simulink model "sldemo_flipflop"  (R2019b)
settings: Solver=VariableStepDiscrete  StartTime=0.0  StopTime=100  RelTol=1e-3  AbsTol=1e-6
StartFcn:
  | set_param('sldemo_flipflop/Display/Scope','Open','on');
libraries: simulink_extras x3
Description:
  | Modulo-4 Counter Using Flip-Flops
  | 
  | This example shows how to use Flip-Flop blocks (found in the Simulink(R)
  | Extras Library) to implement a Modulo-4 counter. The model takes the output
  | of a Modulo-4 counter and generates a half clock cycle width pulse on every
  | fourth clock pulses. Effectively, it produces a pulse whenever both outputs
  | of the Modulo-4 counter are equal to 1.
settings Model: ExtModeTrigMode=oneshot  ExtModeArmWhenConnect=off  ExtModeAutoUpdateStatusClock=off  Creator=The MathWorks, Inc.  LastModifiedBy=The MathWorks, Inc.
settings SolverCC: AutoScaleAbsTol=off
settings DataIOCC: ExternalInput=[]  InitialState=[]  SaveFormat=Array  SaveOutput=off  SignalLogging=off  SaveTime=off
settings OptimizationCC: BlockReduction=off  InitFltsAndDblsToZero=on  LifeSpan=inf  BufferReusableBoundary=off
settings DebuggingCC: SaveWithParameterizedLinksMsg=none  UnderspecifiedInitializationDetection=Classic  MergeDetectMultiDrivingBlocksExec=none  SignalResolutionControl=TryResolveAllWithWarning  MultiTaskDSMMsg=warning  MultiTaskCondExecSysMsg=none  IntegerOverflowMsg=none  FcnCallInpInsideContextMsg=warning  UnconnectedOutputMsg=none  BusObjectLabelMismatch=none  StateNameClashWarn=warning  SFUnexpectedBacktrackingDiag=warning  SFNoUnconditionalDefaultTransitionDiag=warning  SFExecutionAtInitializationDiag=none  IntegerSaturationMsg=none  ArithmeticOperatorsInVariantConditions=warning
settings HardwareCC: ProdBitPerPointer=32  ProdBitPerSizeT=32  ProdBitPerPtrDiffT=32  ProdLargestAtomicFloat=None  ProdIntDivRoundTo=Undefined  ProdEndianess=Unspecified  ProdWordSize=32  ProdHWDeviceType=32-bit Generic  TargetUnknown=on
settings ModelReferenceCC: PropagateSignalLabelsOutOfModel=off
settings SFSimCC: SimUseLocalCustomCode=off  CustomCodeUndefinedFunction=UseInterfaceOnly
settings RTWCC: Description=Generic Real-Time Target  RTWUseLocalCustomCode=off
settings CodeAppCC: StateflowObjectComments=on
settings GRTTargetCC: TargetFcnLib=ansi_tfl_tmw.mat  TargetLangStandard=C89/C90 (ANSI)  GeneratePreprocessorConditionals=Disable all  CombineOutputUpdateFcns=off  GRTInterface=on
settings ConfigComp: CovMetricSettings=d  CovHtmlReporting=on  CovSaveCumulativeToWorkspaceVar=on  CovSaveSingleToWorkspaceVar=on  CovExternalEMLEnable=off

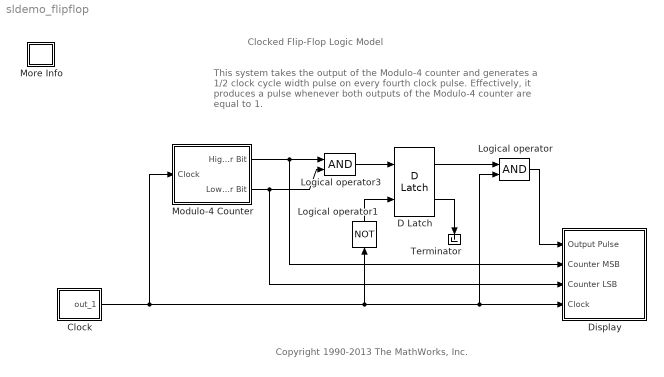
== system sldemo_flipflop ==
  note: This system takes the output of the Modulo-4 counter and
      | generates a 1/2 clock cycle width pulse on every fourth clock pulse.
      | Effectively, it produces a pulse whenever both outputs of the
      | Modulo-4 counter are equal to 1.
  note: Clocked Flip-Flop Logic Model
  note: Copyright 1990-2013 The MathWorks, Inc.
  Clock : Subsystem  mask(BooleanPulseTrain){Period=1}
      mask help:
      | Clock signal for digital logic
      |
      | Output is set to 1 for the first half of the period.
      mask init:
      | onwidth = Period/2;
      mask Help: Digital clock for logic systems.
      mask Display: plot(0,0,100,100,[90,75,75,60,60,35,35,20,20,10],[20,20,80,80,19,20,80,80,20,20])
  D Latch : simulink_extras/Flip Flops/D Latch
      settings: SourceProductName=Simulink  SourceProductBaseCode=SL
  Display : Subsystem
  Logical operator : Logic  IconShape=distinctive
  Logical operator1 : Logic  Operator=NOT  Inputs=1  IconShape=distinctive
  Logical operator3 : Logic  IconShape=distinctive
  Modulo-4 Counter : Subsystem
  More Info : Subsystem
      settings: OpenFcn=showExample('simulink_general/sldemo_flipflopExample')
      mask Display: disp('?')
  Terminator : Terminator
  wires:
  Logical operator3/1 -> D Latch/1
  Logical operator1/1 -> D Latch/2
  D Latch/1 -> Logical operator/1
  Logical operator/1 -> Display/1(Output Pulse)
  Modulo-4 Counter/2(Low-Order Bit) -> Logical operator3/2, Display/3(Counter LSB)
  Modulo-4 Counter/1(High-Order Bit) -> Logical operator3/1, Display/2(Counter MSB)
  D Latch/2 -> Terminator/1
  Clock/1(out_1) -> Logical operator1/1, Display/4(Clock), Logical operator/2, Modulo-4 Counter/1(Clock)

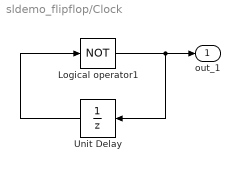
== system sldemo_flipflop/Clock ==
  Logical operator1 : Logic  Operator=NOT  Inputs=1
  Unit Delay : UnitDelay  InitialCondition=boolean(0)  SampleTime=onwidth  HasFrameUpgradeWarning=on
  out_1 : Outport  InitialOutput=0  VectorParamsAs1DForOutWhenUnconnected=off
  wires:
  Logical operator1/1 -> Unit Delay/1, out_1/1
  Unit Delay/1 -> Logical operator1/1

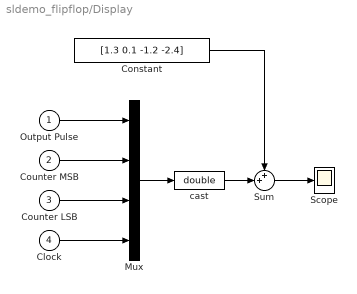
== system sldemo_flipflop/Display ==
  Output Pulse : Inport
  Counter MSB : Inport  Port=2
  Counter LSB : Inport  Port=3
  Clock : Inport  Port=4
  Constant : Constant  Value=[1.3 0.1 -1.2 -2.4]
  Mux : Mux
  Scope : Scope
  Sum : Sum  Inputs=++|  SaturateOnIntegerOverflow=on  InputSameDT=on  OutDataTypeStr=Inherit: Same as first input
  cast : DataTypeConversion  OutDataTypeStr=double  SaturateOnIntegerOverflow=on  RndMeth=Zero
  wires:
  Sum/1 -> Scope/1
  Counter MSB/1 -> Mux/2
  Counter LSB/1 -> Mux/3
  Clock/1 -> Mux/4
  Constant/1 -> Sum/1
  Mux/1 -> cast/1
  Output Pulse/1 -> Mux/1
  cast/1 -> Sum/2

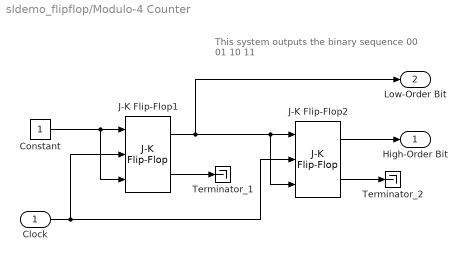
== system sldemo_flipflop/Modulo-4 Counter ==
  note: This system outputs the binary sequence
      | 00 01 10 11
  Clock : Inport
  Constant : Constant  OutDataTypeStr=boolean
  J-K Flip-Flop1 : simulink_extras/Flip Flops/J-K Flip-Flop  initial_condition=0
      settings: SourceProductName=Simulink
  J-K Flip-Flop2 : simulink_extras/Flip Flops/J-K Flip-Flop  initial_condition=0
      settings: SourceProductName=Simulink
  Terminator_1 : Terminator
  Terminator_2 : Terminator
  High-Order Bit : Outport  InitialOutput=0  VectorParamsAs1DForOutWhenUnconnected=off
  Low-Order Bit : Outport  Port=2  InitialOutput=0  VectorParamsAs1DForOutWhenUnconnected=off
  wires:
  J-K Flip-Flop2/2 -> Terminator_2/1
  J-K Flip-Flop1/2 -> Terminator_1/1
  J-K Flip-Flop1/1 -> J-K Flip-Flop2/3, J-K Flip-Flop2/1, Low-Order Bit/1
  Constant/1 -> J-K Flip-Flop1/1, J-K Flip-Flop1/3
  Clock/1 -> J-K Flip-Flop1/2, J-K Flip-Flop2/2
  J-K Flip-Flop2/1 -> High-Order Bit/1

== system sldemo_flipflop/More Info ==
